simulink model "DynamicModel_Cascaded_BAv01"  (R2022b)
settings: Solver=VariableStepAuto  StartTime=0.0  StopTime=9*3600  MaxStep=0.2  RelTol=1e-3
undefined symbols (not defined in the file): driver, getPhysicalConstants, param, route, weatherSim
libraries: slpidlib x5
settings Model: NumberOfSteps=100  Creator=giaco  LastModifiedBy=giaco

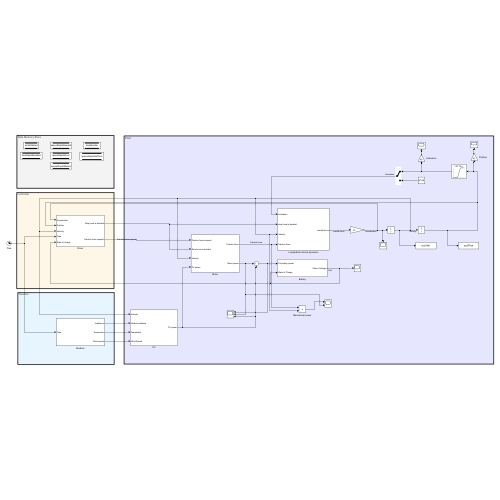
[thumbnail: Simulink's stored preview of the top-level diagram]
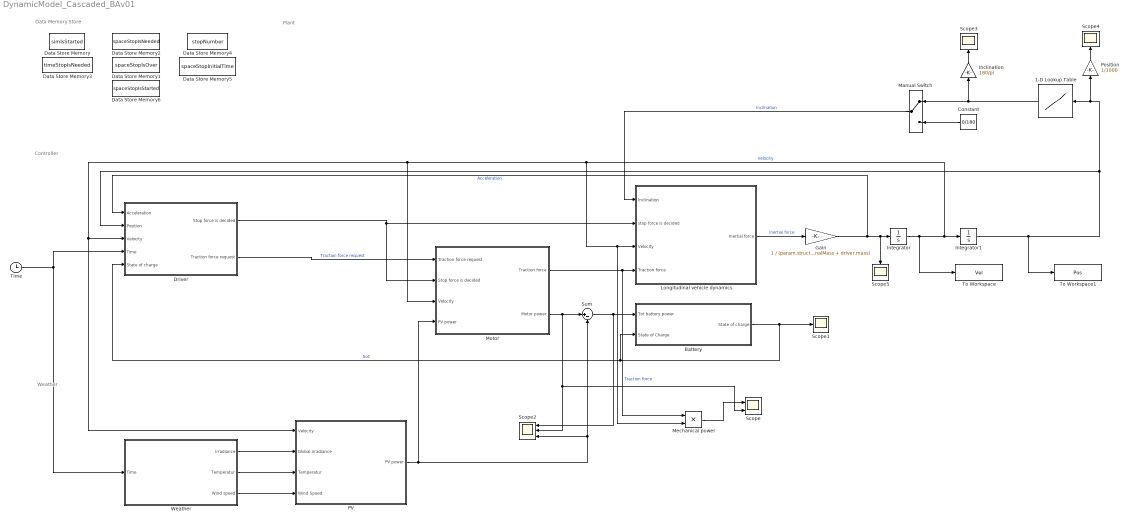
== system DynamicModel_Cascaded_BAv01 ==
  note: Weather
  note: Controller
  note: Plant
  note: Data Memory Store
  1-D Lookup Table : Lookup_n-D  NumberOfTableDimensions=1  BreakpointsForDimension1=route.dist(1:end-1)  Table=route.inclSmooth  InternalRulePriority=Speed  RndMeth=Simplest
  Battery : Subsystem
  Constant : Constant  Value=0/180
  Data Store Memory : DataStoreMemory  DataStoreName=simIsStarted  WriteAfterWriteMsg=warning  InitialValue=1  ShowAdditionalParam=off  OutDataTypeStr=boolean
  Data Store Memory1 : DataStoreMemory  DataStoreName=spaceStopIsOver  WriteAfterWriteMsg=warning  ShowAdditionalParam=off  OutDataTypeStr=boolean
  Data Store Memory2 : DataStoreMemory  DataStoreName=spaceStopIsNeeded  WriteAfterWriteMsg=warning  ShowAdditionalParam=off  OutDataTypeStr=boolean
  Data Store Memory3 : DataStoreMemory  DataStoreName=timeStopIsNeeded  WriteAfterWriteMsg=warning  ShowAdditionalParam=off  OutDataTypeStr=boolean
  Data Store Memory4 : DataStoreMemory  DataStoreName=stopNumber  WriteAfterWriteMsg=warning  InitialValue=2  VectorParams1D=off  ShowAdditionalParam=off  OutDataTypeStr=int8
  Data Store Memory5 : DataStoreMemory  DataStoreName=spaceStopInitialTime  WriteAfterWriteMsg=warning  VectorParams1D=off  ShowAdditionalParam=off  OutDataTypeStr=double
  Data Store Memory6 : DataStoreMemory  DataStoreName=spaceStopIsStarted  WriteAfterWriteMsg=warning  ShowAdditionalParam=off  OutDataTypeStr=boolean
  Driver : Subsystem
  Gain : Gain  Gain=1 / (param.structure.mass + param.motor.rotationalMass + driver.mass)
  Inclination : Gain  Gain=180/pi
  Integrator : Integrator
  Integrator1 : Integrator
  Longitudinal vehicle dynamics : Subsystem
  Manual Switch : ManualSwitch
  Mechanical power : Product
  Motor : Subsystem
  PV : Subsystem
  Position : Gain  Gain=1/1000
  Scope : Scope  NumInputPorts=2
  Scope{1,3..5} (4 alike) : Scope
  Scope2 : Scope  NumInputPorts=3
  Sum : Sum  Inputs=|+-
  Time : Clock
  To Workspace : ToWorkspace  VariableName=Vel  SaveFormat=Timeseries  SampleTime=-1
  To Workspace1 : ToWorkspace  VariableName=Pos  SaveFormat=Timeseries  SampleTime=-1
  Weather : Subsystem
  wires:
  Longitudinal vehicle dynamics/1(Inertial force) -> Gain/1  "Inertial force"
  Gain/1 -> Integrator/1, Scope5/1, Driver/1(Acceleration)  "Acceleration"
  Integrator/1 -> Integrator1/1, Mechanical power/2, Longitudinal vehicle dynamics/3(Velocity), Motor/3(Velocity), PV/1(Velocity), Driver/3(Velocity), To Workspace/1  "Velocity"
  Motor/1(Traction force) -> Mechanical power/1, Longitudinal vehicle dynamics/4(Traction force)  "Traction force"
  Integrator1/1 -> To Workspace1/1, Position/1, 1-D Lookup Table/1, Driver/2(Position)
  1-D Lookup Table/1 -> Inclination/1, Manual Switch/1
  Constant/1 -> Manual Switch/2
  Manual Switch/1 -> Longitudinal vehicle dynamics/1(Inclination)  "Inclination"
  Driver/2(Traction force request) -> Motor/1(Traction force request)  "Traction force request"
  Sum/1 -> Scope2/1, Battery/1(Tot battery power)
  Motor/2(Motor power) -> Scope/2, Scope2/2, Sum/1
  PV/1(PV power) -> Sum/2, Scope2/3, Motor/4(PV power)
  Weather/1(Irradiance) -> PV/2(Global irradiance)
  Weather/2(Temperatur) -> PV/3(Temperatur)
  Weather/3(Wind speed) -> PV/4(Wind Speed)
  Battery/1(State of charge) -> Driver/5(State of charge), Battery/2(State of Charge), Scope1/1  "SoC"
  Position/1 -> Scope4/1
  Inclination/1 -> Scope3/1
  Time/1 -> Weather/1(Time), Driver/4(Time)
  Driver/1(Stop force is decided) -> Motor/2(Stop force is decided), Longitudinal vehicle dynamics/2(stop force is decided)
  Mechanical power/1 -> Scope/1

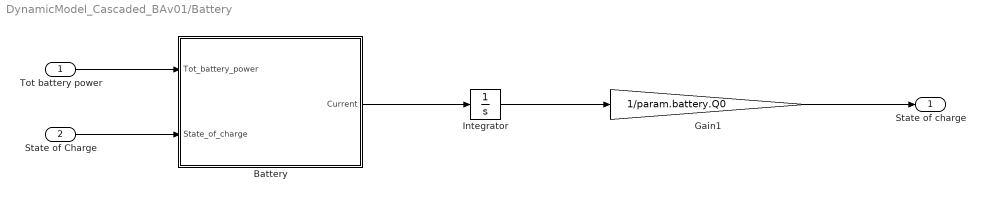
== system DynamicModel_Cascaded_BAv01/Battery ==
  Tot battery power : Inport
  State of Charge : Inport  Port=2
  Battery : MATLAB Function  TreatAsAtomicUnit=on
  Gain1 : Gain  Gain=1/param.battery.Q0
  Integrator : Integrator  InitialCondition=param.battery.Q0
  State of charge : Outport
  wires:
  State of Charge/1 -> Battery/2(State_of_charge)
  Battery/1(Current) -> Integrator/1
  Integrator/1 -> Gain1/1
  Gain1/1 -> State of charge/1
  Tot battery power/1 -> Battery/1(Tot_battery_power)

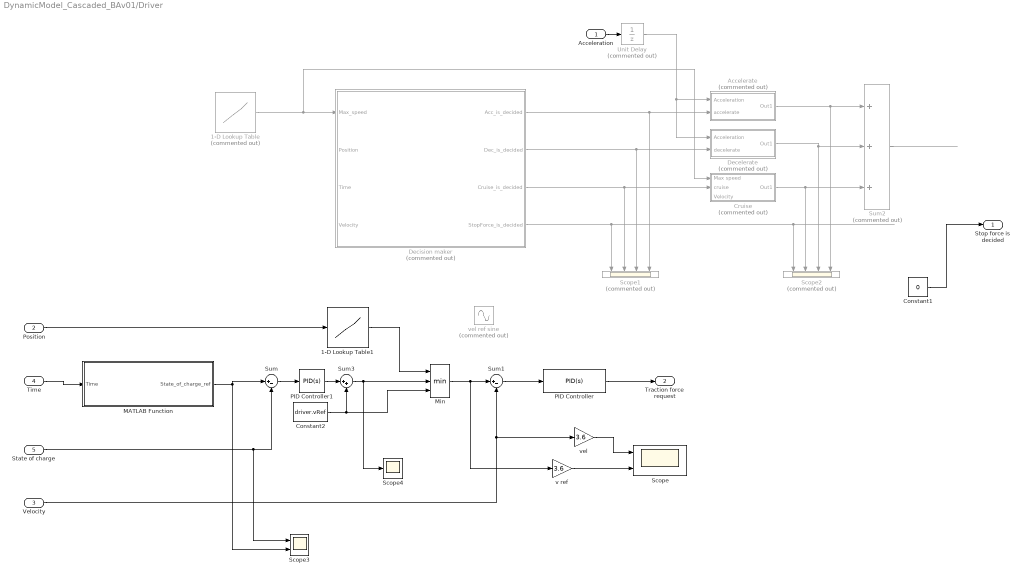
== system DynamicModel_Cascaded_BAv01/Driver ==
  Acceleration : Inport
  Position : Inport  Port=2
  Velocity : Inport  Port=3
  Time : Inport  Port=4
  State of charge : Inport  Port=5
  1-D Lookup Table : Lookup_n-D  Commented=on  NumberOfTableDimensions=1  BreakpointsForDimension1=route.dist  Table=route.maxSpeed  InternalRulePriority=Speed  RndMeth=Simplest
  1-D Lookup Table1 : Lookup_n-D  NumberOfTableDimensions=1  BreakpointsForDimension1=route.dist  Table=route.maxSpeed  InternalRulePriority=Speed  RndMeth=Simplest
  Accelerate : Subsystem  Commented=on
  Constant1 : Constant  Value=0
  Constant2 : Constant  Value=driver.vRef
  Cruise : Subsystem  Commented=on
  Decelerate : Subsystem  Commented=on
  Decision maker : MATLAB Function  Commented=on  TreatAsAtomicUnit=on
  MATLAB Function : MATLAB Function  TreatAsAtomicUnit=on
  Min : MinMax  Inputs=3
  PID Controller : slpidlib/PID Controller  Controller=PID  Form=Parallel  TimeDomain=Continuous-time  UseExternalTs=off  SampleTime=-1  IntegratorMethod=Forward Euler  FilterMethod=Forward Euler  ControllerParametersSource=internal  P=80  I=1  UseKiTs=off  D=0  N=100  UseFilter=on  TunerSelectOption=Transfer Function Based (PID Tuner App)  InitialConditionSource=internal  InitialConditionForIntegrator=0  InitialConditionForFilter=0  DifferentiatorICPrevScaledInput=0  ExternalReset=none  TrackingMode=off  Kt=1  LimitOutput=on  SatLimitsSource=internal  UpperSaturationLimit=param.motor.maxTorque * param.motor.transmissionRatio / param.suspension.rWheel  LowerSaturationLimit=param.motor.minTorque * param.motor.transmissionRatio / param.suspension.rWheel  LinearizeAsGain=on  AntiWindupMode=none  Kb=1  LimitIntegrator=off  UpperIntegratorSaturationLimit=inf  LowerIntegratorSaturationLimit=-inf  POutMin=[]  POutMax=[]  IOutMin=[]  IOutMax=[]  DOutMin=[]  DOutMax=[]  NOutMin=[]  NOutMax=[]  SumOutMin=[]  SumOutMax=[]  SaturationOutMin=[]  SaturationOutMax=[]  PParamMin=[]  PParamMax=[]  IParamMin=[]  IParamMax=[]  DParamMin=[]  DParamMax=[]  NParamMin=[]  NParamMax=[]  KbParamMin=[]  KbParamMax=[]  KtParamMin=[]  KtParamMax=[]  KbOutMin=[]  KbOutMax=[]  KtOutMin=[]  KtOutMax=[]  IntegratorOutMin=[]  IntegratorOutMax=[]  FilterOutMin=[]  FilterOutMax=[]  SumI1OutMin=[]  SumI1OutMax=[]  SumI2OutMin=[]  SumI2OutMax=[]  SumI3OutMin=[]  SumI3OutMax=[]  SumI4OutMin=[]  SumI4OutMax=[]  SumDOutMin=[]  SumDOutMax=[]  DifferentiatorOutMin=[]  DifferentiatorOutMax=[]  FilterDiffOutCoefMin=[]  FilterDiffOutCoefMax=[]  ReciprocalOutMin=[]  ReciprocalOutMax=[]  SumDenOutMin=[]  SumDenOutMax=[]  SumNumOutMin=[]  SumNumOutMax=[]  DivideOutMin=[]  DivideOutMax=[]  UdiffTsProdOutMin=[]  UdiffTsProdOutMax=[]  NTsProdOutMin=[]  NTsProdOutMax=[]  UintegralTsProdOutMin=[]  UintegralTsProdOutMax=[]  UngainTsProdOutMin=[]  UngainTsProdOutMax=[]  ClampingZeroOutDataTypeStr=Inherit: Inherit via back propagation  ClampingZeroOutMin=[]  ClampingZeroOutMax=[]  FilterDenConstantOutDataTypeStr=Inherit: Inherit via back propagation  FilterDenConstantOutMin=[]  FilterDenConstantOutMax=[]  PCopyOutDataTypeStr=Inherit: Inherit via back propagation  PCopyOutMin=[]  PCopyOutMax=[]  NCopyOutDataTypeStr=Inherit: Inherit via back propagation  NCopyOutMin=[]  NCopyOutMax=[]  IntegratorContinuousStateAttributes=''  IntegratorStateMustResolveToSignalObject=off  IntegratorRTWStateStorageClass=Auto  FilterContinuousStateAttributes=''  FilterStateMustResolveToSignalObject=off  FilterRTWStateStorageClass=Auto  ParallelPVariant=InternalParameters  IdealPVariant=Disabled  IVariant=InternalParameters  DVariant=InternalParameters  IntegratorVariant=Continuous  SatVariant=Enabled  AWVariant=Passthrough  PCopyVariant=Disabled  TRVariant=Disabled  FdbkBlocksVariant=Forward  IdealPFdbkVariant=Disabled  SatFdbkVariant=Disabled  DerivativeFilterVariant=ContFilter  NVariant=InternalParameters  NCopyVariant=Disabled  FilterICVariant=InternalICsFilter  IntegratorICVariant=InternalICs  ExternalResetVariant=Disabled  TRSumVariant=Passthrough  SumFdbkVariant=Disabled  SumVariant=Sum_PID  TsampFilterVariant=InternalTs  TsampNgainVariant=Passthrough  TsampIntegralVariant=Passthrough  ExternalSaturationOutDataTypeStr=Inherit: Same as second input
  PID Controller1 : slpidlib/PID Controller  Controller=PID  Form=Ideal  TimeDomain=Continuous-time  UseExternalTs=off  SampleTime=-1  IntegratorMethod=Forward Euler  FilterMethod=Forward Euler  ControllerParametersSource=internal  P=-500  I=1/600  UseKiTs=off  D=0  N=100  UseFilter=on  TunerSelectOption=Transfer Function Based (PID Tuner App)  InitialConditionSource=internal  InitialConditionForIntegrator=0  InitialConditionForFilter=0  DifferentiatorICPrevScaledInput=0  ExternalReset=none  TrackingMode=off  Kt=1  LimitOutput=on  SatLimitsSource=internal  UpperSaturationLimit=inf  LowerSaturationLimit=-driver.vRef*0.9  LinearizeAsGain=on  AntiWindupMode=none  Kb=1  LimitIntegrator=off  UpperIntegratorSaturationLimit=inf  LowerIntegratorSaturationLimit=-inf  POutMin=[]  POutMax=[]  IOutMin=[]  IOutMax=[]  DOutMin=[]  DOutMax=[]  NOutMin=[]  NOutMax=[]  SumOutMin=[]  SumOutMax=[]  SaturationOutMin=[]  SaturationOutMax=[]  PParamMin=[]  PParamMax=[]  IParamMin=[]  IParamMax=[]  DParamMin=[]  DParamMax=[]  NParamMin=[]  NParamMax=[]  KbParamMin=[]  KbParamMax=[]  KtParamMin=[]  KtParamMax=[]  KbOutMin=[]  KbOutMax=[]  KtOutMin=[]  KtOutMax=[]  IntegratorOutMin=[]  IntegratorOutMax=[]  FilterOutMin=[]  FilterOutMax=[]  SumI1OutMin=[]  SumI1OutMax=[]  SumI2OutMin=[]  SumI2OutMax=[]  SumI3OutMin=[]  SumI3OutMax=[]  SumI4OutMin=[]  SumI4OutMax=[]  SumDOutMin=[]  SumDOutMax=[]  DifferentiatorOutMin=[]  DifferentiatorOutMax=[]  FilterDiffOutCoefMin=[]  FilterDiffOutCoefMax=[]  ReciprocalOutMin=[]  ReciprocalOutMax=[]  SumDenOutMin=[]  SumDenOutMax=[]  SumNumOutMin=[]  SumNumOutMax=[]  DivideOutMin=[]  DivideOutMax=[]  UdiffTsProdOutMin=[]  UdiffTsProdOutMax=[]  NTsProdOutMin=[]  NTsProdOutMax=[]  UintegralTsProdOutMin=[]  UintegralTsProdOutMax=[]  UngainTsProdOutMin=[]  UngainTsProdOutMax=[]  ClampingZeroOutDataTypeStr=Inherit: Inherit via back propagation  ClampingZeroOutMin=[]  ClampingZeroOutMax=[]  FilterDenConstantOutDataTypeStr=Inherit: Inherit via back propagation  FilterDenConstantOutMin=[]  FilterDenConstantOutMax=[]  PCopyOutDataTypeStr=Inherit: Inherit via back propagation  PCopyOutMin=[]  PCopyOutMax=[]  NCopyOutDataTypeStr=Inherit: Inherit via back propagation  NCopyOutMin=[]  NCopyOutMax=[]  IntegratorContinuousStateAttributes=''  IntegratorStateMustResolveToSignalObject=off  IntegratorRTWStateStorageClass=Auto  FilterContinuousStateAttributes=''  FilterStateMustResolveToSignalObject=off  FilterRTWStateStorageClass=Auto  ParallelPVariant=Passthrough  IdealPVariant=InternalParameters  IVariant=InternalParameters  DVariant=InternalParameters  IntegratorVariant=Continuous  SatVariant=Enabled  AWVariant=Passthrough  PCopyVariant=Disabled  TRVariant=Disabled  FdbkBlocksVariant=Forward  IdealPFdbkVariant=Disabled  SatFdbkVariant=Disabled  DerivativeFilterVariant=ContFilter  NVariant=InternalParameters  NCopyVariant=Disabled  FilterICVariant=InternalICsFilter  IntegratorICVariant=InternalICs  ExternalResetVariant=Disabled  TRSumVariant=Passthrough  SumFdbkVariant=Disabled  SumVariant=Sum_PID  TsampFilterVariant=InternalTs  TsampNgainVariant=Passthrough  TsampIntegralVariant=Passthrough  ExternalSaturationOutDataTypeStr=Inherit: Same as second input
  Scope : Scope  NumInputPorts=2
  Scope1 : Scope  Commented=on  NumInputPorts=4
  Scope2 : Scope  Commented=on  NumInputPorts=4
  Scope3 : Scope  NumInputPorts=2
  Scope4 : Scope
  Sum : Sum  Inputs=|+-
  Sum1 : Sum  Inputs=|+-
  Sum2 : Sum  Commented=on  Inputs=+++
  Sum3 : Sum  Inputs=|++
  Unit Delay : UnitDelay  Commented=on  SampleTime=-1  HasFrameUpgradeWarning=on
  v ref : Gain  Gain=3.6
  vel : Gain  Gain=3.6
  vel ref sine : Sin  Commented=on  Amplitude=5  Bias=20  Frequency=1/120  SampleTime=0
  Stop force is decided : Outport
  Traction force request : Outport  Port=2
  wires:
  1-D Lookup Table/1 -> Cruise/1(Max speed), Decision maker/1(Max_speed)
  ? -> Decision maker/3(Time)
  Sum2/1 -> ?
  Decision maker/1(Acc_is_decided) -> Accelerate/2(accelerate), Scope1/4
  Acceleration/1 -> Unit Delay/1
  Accelerate/1(Out1) -> Sum2/1, Scope2/4
  Decision maker/2(Dec_is_decided) -> Decelerate/2(decelerate), Scope1/3
  Decelerate/1(Out1) -> Sum2/2, Scope2/3
  Decision maker/3(Cruise_is_decided) -> Scope1/2, Cruise/2(cruise)
  Cruise/1(Out1) -> Sum2/3, Scope2/2
  Unit Delay/1 -> Decelerate/1(Acceleration), Accelerate/1(Acceleration)
  Decision maker/4(StopForce_is_decided) -> Scope1/1, Scope2/1
  ? -> 1-D Lookup Table/1, Decision maker/2(Position)
  ? -> Cruise/3(Velocity), Decision maker/4(Velocity)
  MATLAB Function/1(State_of_charge_ref) -> Sum/1, Scope3/2
  State of charge/1 -> Sum/2, Scope3/1
  Sum/1 -> PID Controller1/1
  Sum1/1 -> PID Controller/1
  Constant1/1 -> Stop force is decided/1
  PID Controller/1 -> Traction force request/1
  Time/1 -> MATLAB Function/1(Time)
  Velocity/1 -> Sum1/2, vel/1
  1-D Lookup Table1/1 -> Min/1
  Position/1 -> 1-D Lookup Table1/1
  v ref/1 -> Scope/2
  vel/1 -> Scope/1
  Min/1 -> v ref/1, Sum1/1
  PID Controller1/1 -> Sum3/1
  Sum3/1 -> Scope4/1, Min/2
  Constant2/1 -> Sum3/2, Min/3

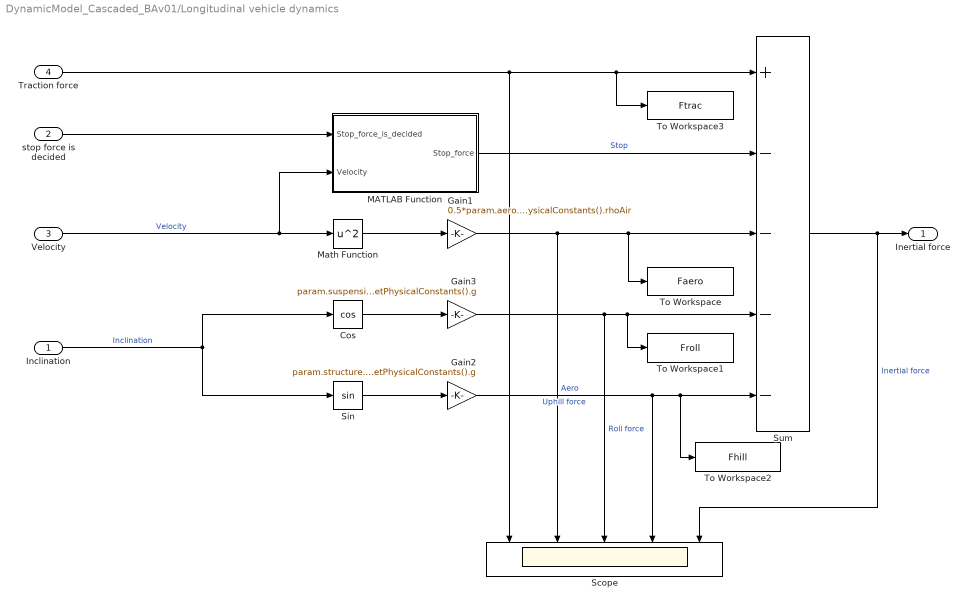
== system DynamicModel_Cascaded_BAv01/Longitudinal vehicle dynamics ==
  Inclination : Inport
  stop force is decided : Inport  Port=2
  Velocity : Inport  Port=3
  Traction force : Inport  Port=4
  Cos : Trigonometry  Operator=cos
  Gain1 : Gain  Gain=0.5*param.aero.AfCd*getPhysicalConstants().rhoAir
  Gain2 : Gain  Gain=param.structure.mass*getPhysicalConstants().g
  Gain3 : Gain  Gain=param.suspension.cR*param.structure.mass*getPhysicalConstants().g
  MATLAB Function : MATLAB Function  TreatAsAtomicUnit=on
  Math Function : Math  Operator=square
  Scope : Scope  NumInputPorts=5
  Sin : Trigonometry
  Sum : Sum  Inputs=+----
  To Workspace : ToWorkspace  VariableName=Faero  SaveFormat=Timeseries  SampleTime=-1
  To Workspace1 : ToWorkspace  VariableName=Froll  SaveFormat=Timeseries  SampleTime=-1
  To Workspace2 : ToWorkspace  VariableName=Fhill  SaveFormat=Timeseries  SampleTime=-1
  To Workspace3 : ToWorkspace  VariableName=Ftrac  SaveFormat=Timeseries  SampleTime=-1
  Inertial force : Outport
  wires:
  Traction force/1 -> To Workspace3/1, Sum/1, Scope/1
  Gain1/1 -> To Workspace/1, Sum/3, Scope/2  "Aero"
  Gain3/1 -> To Workspace1/1, Sum/4, Scope/3  "Roll force"
  Cos/1 -> Gain3/1
  Math Function/1 -> Gain1/1
  Inclination/1 -> Cos/1, Sin/1  "Inclination"
  Sin/1 -> Gain2/1
  Gain2/1 -> To Workspace2/1, Sum/5, Scope/4  "Uphill force"
  Velocity/1 -> MATLAB Function/2(Velocity), Math Function/1  "Velocity"
  Sum/1 -> Inertial force/1, Scope/5  "Inertial force"
  MATLAB Function/1(Stop_force) -> Sum/2  "Stop"
  stop force is decided/1 -> MATLAB Function/1(Stop_force_is_decided)

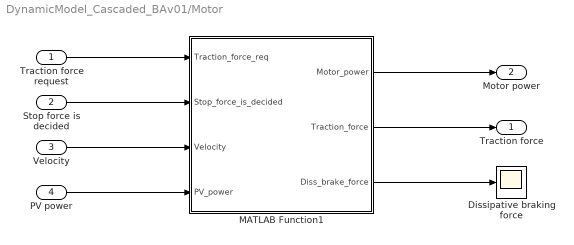
== system DynamicModel_Cascaded_BAv01/Motor ==
  Traction force request : Inport
  Stop force is decided : Inport  Port=2
  Velocity : Inport  Port=3
  PV power : Inport  Port=4
  Dissipative braking force : Scope
  MATLAB Function1 : MATLAB Function  TreatAsAtomicUnit=on
  Traction force : Outport
  Motor power : Outport  Port=2
  wires:
  Traction force request/1 -> MATLAB Function1/1(Traction_force_req)
  Velocity/1 -> MATLAB Function1/3(Velocity)
  MATLAB Function1/1(Motor_power) -> Motor power/1
  MATLAB Function1/2(Traction_force) -> Traction force/1
  MATLAB Function1/3(Diss_brake_force) -> Dissipative braking force/1
  PV power/1 -> MATLAB Function1/4(PV_power)
  Stop force is decided/1 -> MATLAB Function1/2(Stop_force_is_decided)

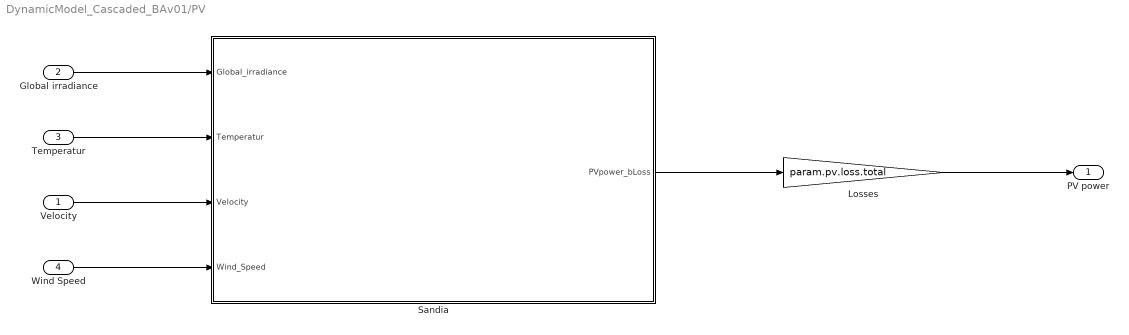
== system DynamicModel_Cascaded_BAv01/PV ==
  Velocity : Inport
  Global irradiance : Inport  Port=2
  Temperatur : Inport  Port=3
  Wind Speed : Inport  Port=4
  Losses : Gain  Gain=param.pv.loss.total
  Sandia : MATLAB Function  TreatAsAtomicUnit=on
  PV power : Outport
  wires:
  Global irradiance/1 -> Sandia/1(Global_irradiance)
  Temperatur/1 -> Sandia/2(Temperatur)
  Sandia/1(PVpower_bLoss) -> Losses/1
  Losses/1 -> PV power/1
  Velocity/1 -> Sandia/3(Velocity)
  Wind Speed/1 -> Sandia/4(Wind_Speed)

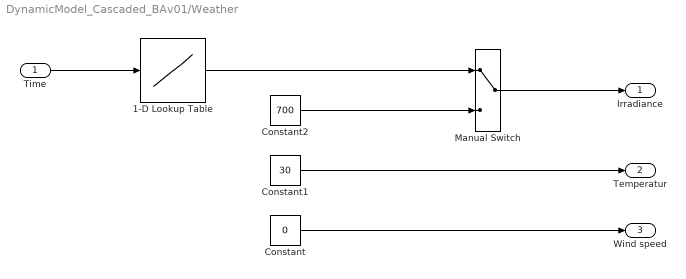
== system DynamicModel_Cascaded_BAv01/Weather ==
  Time : Inport
  1-D Lookup Table : Lookup_n-D  NumberOfTableDimensions=1  BreakpointsForDimension1=weatherSim.timeSec  Table=weatherSim.GtotalSec  InternalRulePriority=Speed  RndMeth=Simplest
  Constant : Constant  Value=0
  Constant1 : Constant  Value=30
  Constant2 : Constant  Value=700
  Manual Switch : ManualSwitch
  Irradiance : Outport
  Temperatur : Outport  Port=2
  Wind speed : Outport  Port=3
  wires:
  Constant1/1 -> Temperatur/1
  Constant2/1 -> Manual Switch/2
  Constant/1 -> Wind speed/1
  Manual Switch/1 -> Irradiance/1
  1-D Lookup Table/1 -> Manual Switch/1
  Time/1 -> 1-D Lookup Table/1

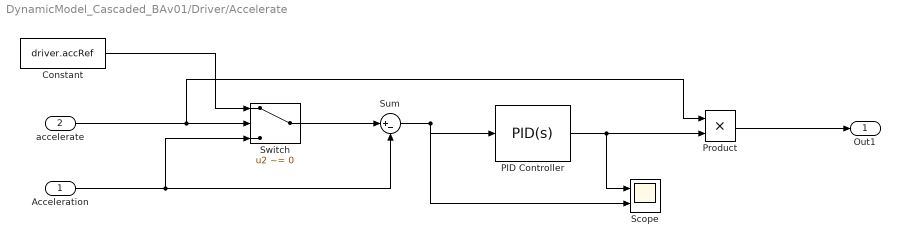
== system DynamicModel_Cascaded_BAv01/Driver/Accelerate ==
  Acceleration : Inport
  accelerate : Inport  Port=2
  Constant : Constant  Value=driver.accRef
  PID Controller : slpidlib/PID Controller  Controller=PID  Form=Parallel  TimeDomain=Continuous-time  UseExternalTs=off  SampleTime=-1  IntegratorMethod=Forward Euler  FilterMethod=Forward Euler  ControllerParametersSource=internal  P=100  I=0  UseKiTs=off  D=0  N=100  UseFilter=on  TunerSelectOption=Transfer Function Based (PID Tuner App)  InitialConditionSource=internal  InitialConditionForIntegrator=0  InitialConditionForFilter=0  DifferentiatorICPrevScaledInput=0  ExternalReset=none  TrackingMode=off  Kt=1  LimitOutput=on  SatLimitsSource=internal  UpperSaturationLimit=param.motor.maxTorque * param.motor.transmissionRatio / param.suspension.rWheel  LowerSaturationLimit=param.motor.minTorque * param.motor.transmissionRatio / param.suspension.rWheel  LinearizeAsGain=on  AntiWindupMode=none  Kb=1  LimitIntegrator=off  UpperIntegratorSaturationLimit=inf  LowerIntegratorSaturationLimit=-inf  POutMin=[]  POutMax=[]  IOutMin=[]  IOutMax=[]  DOutMin=[]  DOutMax=[]  NOutMin=[]  NOutMax=[]  SumOutMin=[]  SumOutMax=[]  SaturationOutMin=[]  SaturationOutMax=[]  PParamMin=[]  PParamMax=[]  IParamMin=[]  IParamMax=[]  DParamMin=[]  DParamMax=[]  NParamMin=[]  NParamMax=[]  KbParamMin=[]  KbParamMax=[]  KtParamMin=[]  KtParamMax=[]  KbOutMin=[]  KbOutMax=[]  KtOutMin=[]  KtOutMax=[]  IntegratorOutMin=[]  IntegratorOutMax=[]  FilterOutMin=[]  FilterOutMax=[]  SumI1OutMin=[]  SumI1OutMax=[]  SumI2OutMin=[]  SumI2OutMax=[]  SumI3OutMin=[]  SumI3OutMax=[]  SumI4OutMin=[]  SumI4OutMax=[]  SumDOutMin=[]  SumDOutMax=[]  DifferentiatorOutMin=[]  DifferentiatorOutMax=[]  FilterDiffOutCoefMin=[]  FilterDiffOutCoefMax=[]  ReciprocalOutMin=[]  ReciprocalOutMax=[]  SumDenOutMin=[]  SumDenOutMax=[]  SumNumOutMin=[]  SumNumOutMax=[]  DivideOutMin=[]  DivideOutMax=[]  UdiffTsProdOutMin=[]  UdiffTsProdOutMax=[]  NTsProdOutMin=[]  NTsProdOutMax=[]  UintegralTsProdOutMin=[]  UintegralTsProdOutMax=[]  UngainTsProdOutMin=[]  UngainTsProdOutMax=[]  ClampingZeroOutDataTypeStr=Inherit: Inherit via back propagation  ClampingZeroOutMin=[]  ClampingZeroOutMax=[]  FilterDenConstantOutDataTypeStr=Inherit: Inherit via back propagation  FilterDenConstantOutMin=[]  FilterDenConstantOutMax=[]  PCopyOutDataTypeStr=Inherit: Inherit via back propagation  PCopyOutMin=[]  PCopyOutMax=[]  NCopyOutDataTypeStr=Inherit: Inherit via back propagation  NCopyOutMin=[]  NCopyOutMax=[]  IntegratorContinuousStateAttributes=''  IntegratorStateMustResolveToSignalObject=off  IntegratorRTWStateStorageClass=Auto  FilterContinuousStateAttributes=''  FilterStateMustResolveToSignalObject=off  FilterRTWStateStorageClass=Auto  ParallelPVariant=InternalParameters  IdealPVariant=Disabled  IVariant=InternalParameters  DVariant=InternalParameters  IntegratorVariant=Continuous  SatVariant=Enabled  AWVariant=Passthrough  PCopyVariant=Disabled  TRVariant=Disabled  FdbkBlocksVariant=Forward  IdealPFdbkVariant=Disabled  SatFdbkVariant=Disabled  DerivativeFilterVariant=ContFilter  NVariant=InternalParameters  NCopyVariant=Disabled  FilterICVariant=InternalICsFilter  IntegratorICVariant=InternalICs  ExternalResetVariant=Disabled  TRSumVariant=Passthrough  SumFdbkVariant=Disabled  SumVariant=Sum_PID  TsampFilterVariant=InternalTs  TsampNgainVariant=Passthrough  TsampIntegralVariant=Passthrough  ExternalSaturationOutDataTypeStr=Inherit: Same as second input
  Product : Product
  Scope : Scope  NumInputPorts=2
  Sum : Sum  Inputs=|+-
  Switch : Switch  Criteria=u2 ~= 0  SaturateOnIntegerOverflow=off  InputSameDT=off
  Out1 : Outport
  wires:
  accelerate/1 -> Product/1, Switch/2
  Constant/1 -> Switch/1
  Switch/1 -> Sum/1
  Acceleration/1 -> Sum/2, Switch/3
  Sum/1 -> Scope/2, PID Controller/1
  PID Controller/1 -> Product/2, Scope/1
  Product/1 -> Out1/1

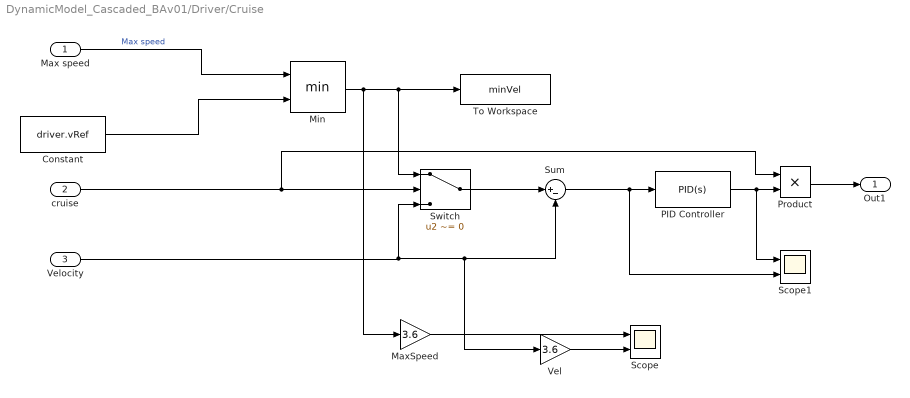
== system DynamicModel_Cascaded_BAv01/Driver/Cruise ==
  Max speed : Inport
  cruise : Inport  Port=2
  Velocity : Inport  Port=3
  Constant : Constant  Value=driver.vRef
  MaxSpeed : Gain  Gain=3.6
  Min : MinMax  Inputs=2
  PID Controller : slpidlib/PID Controller  Controller=PID  Form=Parallel  TimeDomain=Continuous-time  UseExternalTs=off  SampleTime=-1  IntegratorMethod=Forward Euler  FilterMethod=Forward Euler  ControllerParametersSource=internal  P=driver.Pf  I=driver.If  UseKiTs=off  D=driver.Df  N=driver.Nf  UseFilter=on  TunerSelectOption=Transfer Function Based (PID Tuner App)  InitialConditionSource=internal  InitialConditionForIntegrator=0  InitialConditionForFilter=0  DifferentiatorICPrevScaledInput=0  ExternalReset=none  TrackingMode=off  Kt=1  LimitOutput=on  SatLimitsSource=internal  UpperSaturationLimit=param.motor.maxTorque * param.motor.transmissionRatio / param.suspension.rWheel  LowerSaturationLimit=param.motor.minTorque * param.motor.transmissionRatio / param.suspension.rWheel  LinearizeAsGain=on  AntiWindupMode=none  Kb=1  LimitIntegrator=off  UpperIntegratorSaturationLimit=inf  LowerIntegratorSaturationLimit=-inf  POutMin=[]  POutMax=[]  IOutMin=[]  IOutMax=[]  DOutMin=[]  DOutMax=[]  NOutMin=[]  NOutMax=[]  SumOutMin=[]  SumOutMax=[]  SaturationOutMin=[]  SaturationOutMax=[]  PParamMin=[]  PParamMax=[]  IParamMin=[]  IParamMax=[]  DParamMin=[]  DParamMax=[]  NParamMin=[]  NParamMax=[]  KbParamMin=[]  KbParamMax=[]  KtParamMin=[]  KtParamMax=[]  KbOutMin=[]  KbOutMax=[]  KtOutMin=[]  KtOutMax=[]  IntegratorOutMin=[]  IntegratorOutMax=[]  FilterOutMin=[]  FilterOutMax=[]  SumI1OutMin=[]  SumI1OutMax=[]  SumI2OutMin=[]  SumI2OutMax=[]  SumI3OutMin=[]  SumI3OutMax=[]  SumI4OutMin=[]  SumI4OutMax=[]  SumDOutMin=[]  SumDOutMax=[]  DifferentiatorOutMin=[]  DifferentiatorOutMax=[]  FilterDiffOutCoefMin=[]  FilterDiffOutCoefMax=[]  ReciprocalOutMin=[]  ReciprocalOutMax=[]  SumDenOutMin=[]  SumDenOutMax=[]  SumNumOutMin=[]  SumNumOutMax=[]  DivideOutMin=[]  DivideOutMax=[]  UdiffTsProdOutMin=[]  UdiffTsProdOutMax=[]  NTsProdOutMin=[]  NTsProdOutMax=[]  UintegralTsProdOutMin=[]  UintegralTsProdOutMax=[]  UngainTsProdOutMin=[]  UngainTsProdOutMax=[]  ClampingZeroOutDataTypeStr=Inherit: Inherit via back propagation  ClampingZeroOutMin=[]  ClampingZeroOutMax=[]  FilterDenConstantOutDataTypeStr=Inherit: Inherit via back propagation  FilterDenConstantOutMin=[]  FilterDenConstantOutMax=[]  PCopyOutDataTypeStr=Inherit: Inherit via back propagation  PCopyOutMin=[]  PCopyOutMax=[]  NCopyOutDataTypeStr=Inherit: Inherit via back propagation  NCopyOutMin=[]  NCopyOutMax=[]  IntegratorContinuousStateAttributes=''  IntegratorStateMustResolveToSignalObject=off  IntegratorRTWStateStorageClass=Auto  FilterContinuousStateAttributes=''  FilterStateMustResolveToSignalObject=off  FilterRTWStateStorageClass=Auto  ParallelPVariant=InternalParameters  IdealPVariant=Disabled  IVariant=InternalParameters  DVariant=InternalParameters  IntegratorVariant=Continuous  SatVariant=Enabled  AWVariant=Passthrough  PCopyVariant=Disabled  TRVariant=Disabled  FdbkBlocksVariant=Forward  IdealPFdbkVariant=Disabled  SatFdbkVariant=Disabled  DerivativeFilterVariant=ContFilter  NVariant=InternalParameters  NCopyVariant=Disabled  FilterICVariant=InternalICsFilter  IntegratorICVariant=InternalICs  ExternalResetVariant=Disabled  TRSumVariant=Passthrough  SumFdbkVariant=Disabled  SumVariant=Sum_PID  TsampFilterVariant=InternalTs  TsampNgainVariant=Passthrough  TsampIntegralVariant=Passthrough  ExternalSaturationOutDataTypeStr=Inherit: Same as second input
  Product : Product
  Scope : Scope  NumInputPorts=2
  Scope1 : Scope  NumInputPorts=2
  Sum : Sum  Inputs=|+-
  Switch : Switch  Criteria=u2 ~= 0  SaturateOnIntegerOverflow=off  InputSameDT=off
  To Workspace : ToWorkspace  VariableName=minVel  SaveFormat=Timeseries  SampleTime=-1
  Vel : Gain  Gain=3.6
  Out1 : Outport
  wires:
  cruise/1 -> Product/1, Switch/2
  Max speed/1 -> Min/1  "Max speed"
  Min/1 -> MaxSpeed/1, Switch/1, To Workspace/1
  Constant/1 -> Min/2
  Velocity/1 -> Vel/1, Sum/2, Switch/3
  Switch/1 -> Sum/1
  MaxSpeed/1 -> Scope/1
  Vel/1 -> Scope/2
  PID Controller/1 -> Product/2, Scope1/1
  Sum/1 -> Scope1/2, PID Controller/1
  Product/1 -> Out1/1

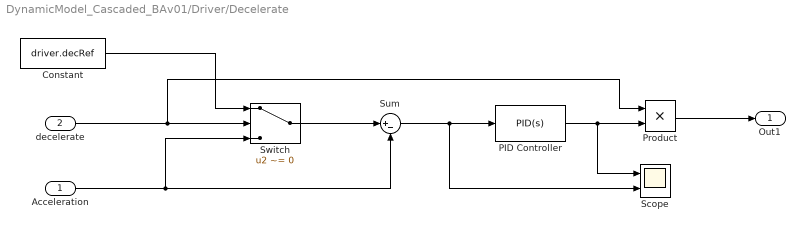
== system DynamicModel_Cascaded_BAv01/Driver/Decelerate ==
  Acceleration : Inport
  decelerate : Inport  Port=2
  Constant : Constant  Value=driver.decRef
  PID Controller : slpidlib/PID Controller  Controller=PID  Form=Parallel  TimeDomain=Continuous-time  UseExternalTs=off  SampleTime=-1  IntegratorMethod=Forward Euler  FilterMethod=Forward Euler  ControllerParametersSource=internal  P=100  I=0  UseKiTs=off  D=0  N=100  UseFilter=on  TunerSelectOption=Transfer Function Based (PID Tuner App)  InitialConditionSource=internal  InitialConditionForIntegrator=0  InitialConditionForFilter=0  DifferentiatorICPrevScaledInput=0  ExternalReset=none  TrackingMode=off  Kt=1  LimitOutput=on  SatLimitsSource=internal  UpperSaturationLimit=param.motor.maxTorque * param.motor.transmissionRatio / param.suspension.rWheel  LowerSaturationLimit=param.motor.minTorque * param.motor.transmissionRatio / param.suspension.rWheel  LinearizeAsGain=on  AntiWindupMode=none  Kb=1  LimitIntegrator=off  UpperIntegratorSaturationLimit=inf  LowerIntegratorSaturationLimit=-inf  POutMin=[]  POutMax=[]  IOutMin=[]  IOutMax=[]  DOutMin=[]  DOutMax=[]  NOutMin=[]  NOutMax=[]  SumOutMin=[]  SumOutMax=[]  SaturationOutMin=[]  SaturationOutMax=[]  PParamMin=[]  PParamMax=[]  IParamMin=[]  IParamMax=[]  DParamMin=[]  DParamMax=[]  NParamMin=[]  NParamMax=[]  KbParamMin=[]  KbParamMax=[]  KtParamMin=[]  KtParamMax=[]  KbOutMin=[]  KbOutMax=[]  KtOutMin=[]  KtOutMax=[]  IntegratorOutMin=[]  IntegratorOutMax=[]  FilterOutMin=[]  FilterOutMax=[]  SumI1OutMin=[]  SumI1OutMax=[]  SumI2OutMin=[]  SumI2OutMax=[]  SumI3OutMin=[]  SumI3OutMax=[]  SumI4OutMin=[]  SumI4OutMax=[]  SumDOutMin=[]  SumDOutMax=[]  DifferentiatorOutMin=[]  DifferentiatorOutMax=[]  FilterDiffOutCoefMin=[]  FilterDiffOutCoefMax=[]  ReciprocalOutMin=[]  ReciprocalOutMax=[]  SumDenOutMin=[]  SumDenOutMax=[]  SumNumOutMin=[]  SumNumOutMax=[]  DivideOutMin=[]  DivideOutMax=[]  UdiffTsProdOutMin=[]  UdiffTsProdOutMax=[]  NTsProdOutMin=[]  NTsProdOutMax=[]  UintegralTsProdOutMin=[]  UintegralTsProdOutMax=[]  UngainTsProdOutMin=[]  UngainTsProdOutMax=[]  ClampingZeroOutDataTypeStr=Inherit: Inherit via back propagation  ClampingZeroOutMin=[]  ClampingZeroOutMax=[]  FilterDenConstantOutDataTypeStr=Inherit: Inherit via back propagation  FilterDenConstantOutMin=[]  FilterDenConstantOutMax=[]  PCopyOutDataTypeStr=Inherit: Inherit via back propagation  PCopyOutMin=[]  PCopyOutMax=[]  NCopyOutDataTypeStr=Inherit: Inherit via back propagation  NCopyOutMin=[]  NCopyOutMax=[]  IntegratorContinuousStateAttributes=''  IntegratorStateMustResolveToSignalObject=off  IntegratorRTWStateStorageClass=Auto  FilterContinuousStateAttributes=''  FilterStateMustResolveToSignalObject=off  FilterRTWStateStorageClass=Auto  ParallelPVariant=InternalParameters  IdealPVariant=Disabled  IVariant=InternalParameters  DVariant=InternalParameters  IntegratorVariant=Continuous  SatVariant=Enabled  AWVariant=Passthrough  PCopyVariant=Disabled  TRVariant=Disabled  FdbkBlocksVariant=Forward  IdealPFdbkVariant=Disabled  SatFdbkVariant=Disabled  DerivativeFilterVariant=ContFilter  NVariant=InternalParameters  NCopyVariant=Disabled  FilterICVariant=InternalICsFilter  IntegratorICVariant=InternalICs  ExternalResetVariant=Disabled  TRSumVariant=Passthrough  SumFdbkVariant=Disabled  SumVariant=Sum_PID  TsampFilterVariant=InternalTs  TsampNgainVariant=Passthrough  TsampIntegralVariant=Passthrough  ExternalSaturationOutDataTypeStr=Inherit: Same as second input
  Product : Product
  Scope : Scope  NumInputPorts=2
  Sum : Sum  Inputs=|+-
  Switch : Switch  Criteria=u2 ~= 0  SaturateOnIntegerOverflow=off  InputSameDT=off
  Out1 : Outport
  wires:
  decelerate/1 -> Product/1, Switch/2
  Constant/1 -> Switch/1
  Switch/1 -> Sum/1
  Acceleration/1 -> Sum/2, Switch/3
  PID Controller/1 -> Product/2, Scope/1
  Sum/1 -> Scope/2, PID Controller/1
  Product/1 -> Out1/1

== matlab function DynamicModel_Cascaded_BAv01/Driver/MATLAB Function ==
  data: Time input; State_of_charge_ref output; param parameter
function State_of_charge_ref = fcn(Time, param)

% State_of_charge_ref = 1 - 0.5 / (9*3600) * Time;
State_of_charge_ref = param.strategy.a*Time.^2 + param.strategy.b*Time + param.strategy.c;

== matlab function DynamicModel_Cascaded_BAv01/PV/Sandia ==
  data: Global_irradiance input; Temperatur input; Velocity input; PVpower_bLoss output; Wind_Speed input; param parameter
function PVpower_bLoss = fcn(Global_irradiance, Temperatur, Velocity, Wind_Speed, param)

type = "glass-cell-polymer";
mounting = "open rack";

relVelocity = Velocity - Wind_Speed;

switch type
    case "glass-cell-glass"
        if mounting == "open rack"
            a = -3.47;
            b = -0.0594;
            deltaTemp = 3;
        elseif mounting == "close roof mount"
            a = -2.98;
            b = -0.0471;
            deltaTemp = 1;
        end % if
    case "glass-cell-polymer"
        if mounting == "open rack"
            a = -3.56;
            b = -0.075;
            deltaTemp = 3;
        elseif mounting == "insulated back"
            a = -2.81;
            b = -0.0455;
            deltaTemp = 0;
        end % if
    case "polymer-thinfilm-steel"
        if mounting == "open rack"
            a = -3.58;
            b = -0.113;
            deltaTemp = 3;
        end % if
    otherwise
        a = -3.56;
        b = -0.075;
        deltaTemp = 3;
end % switch

tempModule = Global_irradiance.* exp(a + b.*relVelocity) + Temperatur;
tempCell = tempModule + Global_irradiance / param.pv.G0 * deltaTemp;


PVpower_bLoss = param.pv.area * Global_irradiance * param.pv.eff * (1 + param.pv.powerCoeff * (tempCell - param.pv.tempSTC));

== matlab function DynamicModel_Cascaded_BAv01/Battery/Battery ==
  data: Tot_battery_power input; State_of_charge input; Current output; param parameter
function Current = fcn(Tot_battery_power, State_of_charge, param)

%conversion to single battery power
Battery_power = Tot_battery_power ./ param.battery.totNum;

%OC parameters
Uoc = param.battery.k2 .* State_of_charge + param.battery.k1;
Ri = param.battery.k4 .* State_of_charge + param.battery.k3;

%solution of quadratic equation
Current = (Uoc - sqrt(Uoc^2 - 4*Battery_power*Ri)) / (2*Ri);

%Coulomb efficiency
Current = -1 * param.battery.effCoul .* Current;

== matlab function DynamicModel_Cascaded_BAv01/Longitudinal vehicle dynamics/MATLAB Function ==
  data: Stop_force_is_decided input; Velocity input; Stop_force output
function Stop_force = fcn(Stop_force_is_decided, Velocity)

Stop_force = 0;

if Stop_force_is_decided == true
    Stop_force = 100 * sign(Velocity);
end % if

== matlab function DynamicModel_Cascaded_BAv01/Driver/Decision maker ==
  settings: updateMethod=DISCRETE
  data: Max_speed input; Position input; Time input; Velocity input; simIsStarted data_store_memory; spaceStopIsOver data_store_memory; timeStopIsNeeded data_store_memory; spaceStopIsNeeded data_store_memory; driver parameter; stopNumber data_store_memory; spaceStopIsStarted data_store_memory; Acc_is_decided output; Dec_is_decided output; Cruise_is_decided output; StopForce_is_decided output; spaceStopInitialTime data_store_memory
function [Acc_is_decided, Dec_is_decided, Cruise_is_decided, StopForce_is_decided] = fcn(Max_speed, Position, Time, Velocity, driver)

global simIsStarted
global spaceStopIsOver
global timeStopIsNeeded;
global spaceStopIsNeeded;
global spaceStopIsStarted;

global stopNumber;
global spaceStopInitialTime;

Acc_is_decided = false;
Dec_is_decided = false;
Cruise_is_decided = false;
StopForce_is_decided = false;

%% Check for stops
% Time stops
stopTime = Time - Velocity ./ driver.decRef;

%assuming the simulation starts at 08.00 and therefore stops at 17.00
if stopTime >= 9*3600
    timeStopIsNeeded = true;
end % if

% Space stops
stopDistance = Position - Velocity.^2 / (2 * driver.decRef);

if stopDistance >= driver.stopLocDist(stopNumber)
    spaceStopIsNeeded = true;
    stopNumber = stopNumber + 1;
end % if

%% Select control options
controlVelocity = min(driver.vRef, Max_speed);

if simIsStarted || spaceStopIsOver                               % 1. Acceleration
    if  Velocity >= 0.9 * controlVelocity
        Cruise_is_decided = true;
        simIsStarted = false;
        spaceStopIsOver = false;
    else
        Acc_is_decided = true;
    end % if

    
elseif spaceStopIsNeeded                                                % 2. Deceleration
    if spaceStopIsStarted
        spaceStopDuration = Time - spaceStopInitialTime;
        if spaceStopDuration >= 30*60
            spaceStopIsNeeded = false;
            spaceStopIsStarted = false;
            spaceStopIsOver = true;
            StopForce_is_decided = false;
            Acc_is_decided = true;
        else
            StopForce_is_decided = true;
        end % if
    else
        if Velocity > driver.vRefStop
            Dec_is_decided = true;
        elseif Velocity <= driver.vRefStop
            spaceStopIsStarted = true;
            spaceStopInitialTime = Time;
            StopForce_is_decided = true;
        end % if
    end % if


elseif timeStopIsNeeded                                                 % 2. Deceleration
    Dec_is_decided = true;
    %stop simulation?????? TODO
else                                                                        % 3. Cruise velocity
    Cruise_is_decided = true;
end % if

== matlab function DynamicModel_Cascaded_BAv01/Motor/MATLAB Function1 ==
  data: Traction_force_req input; Stop_force_is_decided input; Velocity input; PV_power input; param parameter; Motor_power output; Traction_force output; Diss_brake_force output
function [Motor_power, Traction_force, Diss_brake_force] = fcn(Traction_force_req, Stop_force_is_decided, Velocity, PV_power, param)

Diss_brake_force = 0; %normally


if Stop_force_is_decided
    Traction_force = 0;
    Motor_power = 0;

%condition for standing - avoid division with zero
elseif Velocity == 0
    Motor_power = param.motor.maxPower ./ 5;
    Traction_force = Traction_force_req ./ 5;
else
    
    %% POWER
    %conversion to torque
    tractionTorque = param.suspension.rWheel/param.motor.transmissionRatio .* Traction_force_req;
    %limits on the torque
    tractionTorque = min(tractionTorque, param.motor.maxTorque);
    tractionTorque = max(tractionTorque, param.motor.minTorque);
    
    %conversion to angular velocity
    omega = param.motor.transmissionRatio/param.suspension.rWheel .* Velocity;
    
    
    %mechanical power
    mechPower = omega .* tractionTorque;
    %limits on the power
    maxPowerMotBat = param.battery.maxPowerDelta .* param.battery.totNum + PV_power;
    mechPower = min(mechPower, maxPowerMotBat); %upper limit battery
%     minPowerMotBat = param.battery.minPower .* param.battery.totNum + PV_power;
%     mechPower = max(mechPower, minPowerMotBat); %lower limit battery

    mechPower = min(mechPower, param.motor.maxPower); %upper limit motor
    mechPower = max(mechPower, param.motor.minPower); %lower limit motor
    
    
    %electrical power / motor power
    if mechPower >= 0
        Motor_power = (mechPower + param.motor.p0) / param.motor.efficiency;
    else
        Motor_power = (mechPower + param.motor.p0) * param.motor.efficiency;
    end % if

    %% FORCE
    Traction_force = mechPower ./ Velocity;

    %additional dissapitive braking force
    deltaBrake = Traction_force_req - Traction_force;
    if deltaBrake < 0
        Diss_brake_force = deltaBrake;
        Traction_force = Traction_force + Diss_brake_force;
    end %if
end % if
